simulink model "p7"  (R2020a)
settings: Solver=VariableStepAuto  StartTime=0.0  StopTime=10.0  RelTol=1e-3
model workspace (MAT data in the model file):
  g1 = Simulink.Parameter
  g1.Value = 2
  g1.DataType = 'auto'
  g1.Dimensions = [1 1]
  g2 = Simulink.Parameter
  g2.Value = -1
  g2.DataType = 'auto'
  g2.Dimensions = [1 1]
  g3 = Simulink.Parameter
  g3.Value = 1
  g3.DataType = 'auto'
  g3.Dimensions = [1 1]
  g4 = Simulink.Parameter
  g4.Value = -1
  g4.DataType = 'auto'
  g4.Dimensions = [1 1]
settings Model: Creator=akhil singh  LastModifiedBy=akhil singh

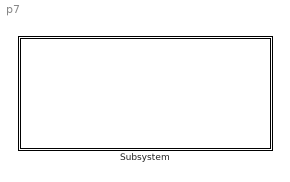
== system p7 ==
  Subsystem : Subsystem

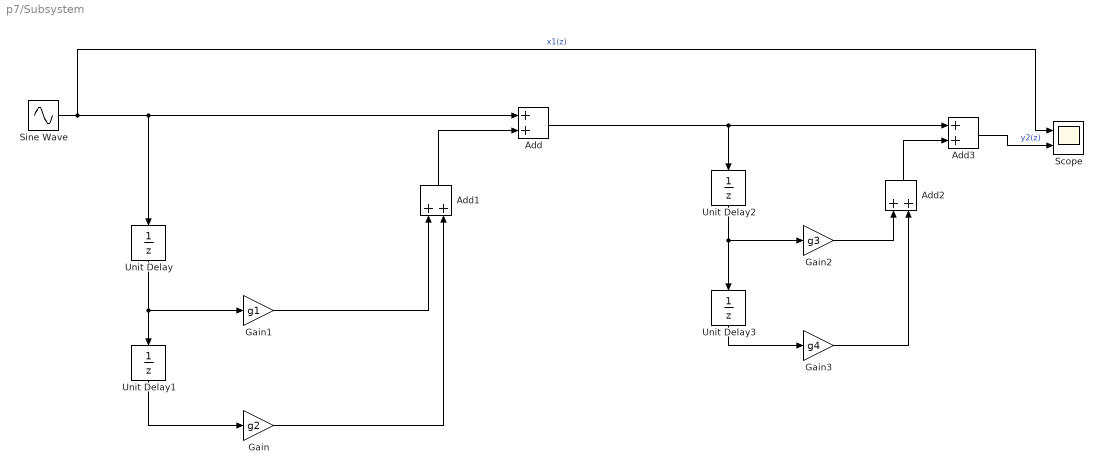
== system p7/Subsystem ==
  Add{,1..3} (4 alike) : Sum
  Gain : Gain  Gain=g2
  Gain1 : Gain  Gain=g1
  Gain2 : Gain  Gain=g3
  Gain3 : Gain  Gain=g4
  Scope : Scope  NumInputPorts=2
  Sine Wave : Sin  SampleTime=0
  Unit Delay{,1..3} (4 alike) : UnitDelay  SampleTime=-1  HasFrameUpgradeWarning=on
  wires:
  Unit Delay/1 -> Gain1/1, Unit Delay1/1
  Sine Wave/1 -> Scope/1, Unit Delay/1, Add/1  "x1(z)"
  Gain/1 -> Add1/2
  Gain3/1 -> Add2/2
  Add/1 -> Unit Delay2/1, Add3/1
  Add3/1 -> Scope/2  "y2(z)"
  Unit Delay2/1 -> Gain2/1, Unit Delay3/1
  Unit Delay1/1 -> Gain/1
  Gain1/1 -> Add1/1
  Gain2/1 -> Add2/1
  Unit Delay3/1 -> Gain3/1
  Add2/1 -> Add3/2
  Add1/1 -> Add/2
